simulink model "SimulacionControladores"  (R2020a)
settings: Solver=VariableStepAuto  StartTime=0.0  StopTime=200  RelTol=1e-3
libraries: simulink x1
settings Model: Creator=mario.giraldo  LastModifiedBy=Julian.Gaona

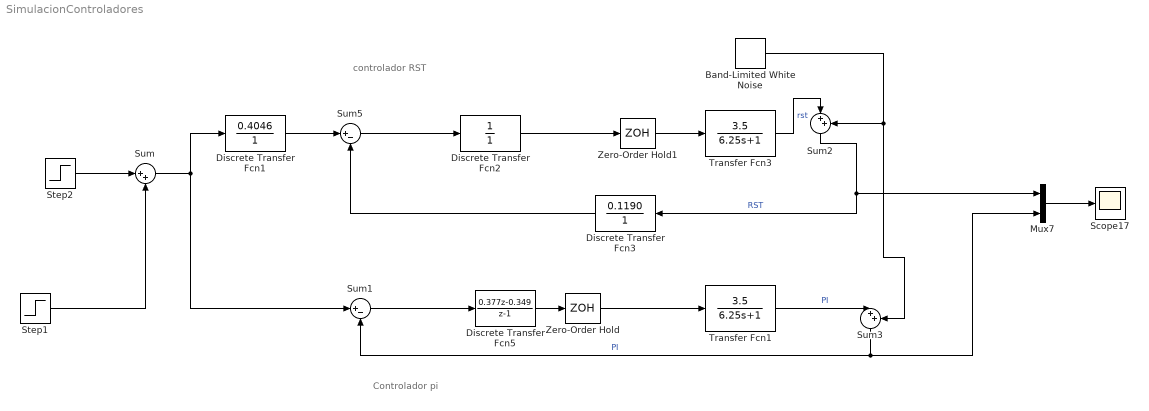
== system SimulacionControladores ==
  note: controlador RST
  note: Controlador pi
  Band-Limited White Noise : simulink/Sources/Band-Limited White Noise  Cov=[0.0000001]  Ts=0.27  seed=[01010]  VectorParams1D=off
  Discrete Transfer Fcn1 : DiscreteTransferFcn  Numerator=[0.4046]  Denominator=[1]
  Discrete Transfer Fcn2 : DiscreteTransferFcn  Denominator=[1]
  Discrete Transfer Fcn3 : DiscreteTransferFcn  Numerator=[0.1190]  Denominator=[1]
  Discrete Transfer Fcn5 : DiscreteTransferFcn  Numerator=[0.377 -0.349]  Denominator=[1 -1]
  Mux7 : Mux  Inputs=2
  Scope17 : Scope
  Step1 : Step  After=20  SampleTime=0
  Step2 : Step  Time=40  After=20  SampleTime=0
  Sum : Sum  Inputs=|++
  Sum1 : Sum  Inputs=|+-
  Sum2 : Sum  Inputs=|++
  Sum3 : Sum  Inputs=|++
  Sum5 : Sum  Inputs=|+-
  Transfer Fcn1 : TransferFcn  Numerator=[3.5]  Denominator=[6.25 1]
  Transfer Fcn3 : TransferFcn  Numerator=[3.5]  Denominator=[6.25 1]
  Zero-Order Hold : ZeroOrderHold  SampleTime=-1
  Zero-Order Hold1 : ZeroOrderHold  SampleTime=-1
  wires:
  Sum5/1 -> Discrete Transfer Fcn2/1
  Mux7/1 -> Scope17/1
  Zero-Order Hold1/1 -> Transfer Fcn3/1
  Discrete Transfer Fcn2/1 -> Zero-Order Hold1/1
  Discrete Transfer Fcn3/1 -> Sum5/2
  Discrete Transfer Fcn1/1 -> Sum5/1
  Discrete Transfer Fcn5/1 -> Zero-Order Hold/1
  Sum1/1 -> Discrete Transfer Fcn5/1
  Zero-Order Hold/1 -> Transfer Fcn1/1
  Step1/1 -> Sum/2
  Sum/1 -> Sum1/1, Discrete Transfer Fcn1/1
  Step2/1 -> Sum/1
  Transfer Fcn3/1 -> Sum2/1  "rst"
  Sum2/1 -> Discrete Transfer Fcn3/1, Mux7/1  "RST"
  Band-Limited White Noise/1 -> Sum3/2, Sum2/2
  Transfer Fcn1/1 -> Sum3/1  "PI"
  Sum3/1 -> Mux7/2, Sum1/2  "PI"
